simulink model "phase1_PRControl_CIM_Adapt"  (R2024a)
settings: Solver=VariableStepAuto  StartTime=0.0  StopTime=20  FixedStep=1e-6  MaxStep=1e-6  RelTol=1e-6
values from neighbouring files (symbols this model uses):
  alpha_adapt = 100    [phase1_PRControl_CIM_Adapt_init.m]
  Am0_can = sys0_ocf.A    [phase1_PRControl_CIM_Adapt_init.m]
  Bm1_can = sys1_ocf.B    [phase1_PRControl_CIM_Adapt_init.m]
  c_adapt = 0.1    [phase1_PRControl_CIM_Adapt_init.m]
  Cf = 22e-6    (= 2.2e-05)    [phase1_PRControl_CIM_Adapt_init.m]
  Cm0_can = sys0_ocf.C    [phase1_PRControl_CIM_Adapt_init.m]
  E = 1    [phase1_PRControl_CIM_Adapt_init.m]
  freq = 49.5    [phase1_PRControl_CIM_Adapt_init.m]
  L1 = 150e-6    (= 0.00015)    [phase1_PRControl_CIM_Adapt_init.m]
  L2g = L2+Lg    (= 0.00045)    [phase1_PRControl_CIM_Adapt_init.m]
  m_m1 = size(Bm1_can,2)    [phase1_PRControl_CIM_Adapt_init.m]
  n_m0 = size(Am0_can,1)    [phase1_PRControl_CIM_Adapt_init.m]
  p_e = size(E,1)    [phase1_PRControl_CIM_Adapt_init.m]
  PiInit = k0_adapt*eye(m_m1)    [phase1_PRControl_CIM_Adapt_init.m]
  Q_adapt = zeros(m_m1,1)    [phase1_PRControl_CIM_Adapt_init.m]
  R1 = 0.045    [phase1_PRControl_CIM_Adapt_init.m]
  R2g = R2+Rg    (= 0.135)    [phase1_PRControl_CIM_Adapt_init.m]
  Rd = 1    [phase1_PRControl_CIM_Adapt_init.m]
  Theta0 = w0^2    (= 98696.0440109)    [phase1_PRControl_CIM_Adapt_init.m]
  w = 2*pi*freq    (= 311.017672705)    [phase1_PRControl_CIM_Adapt_init.m]
undefined symbols (not defined in the file or in its folder): alfa, Am0, beta, Bm1, C_filter, Cm1, DiscIntNeverNeededParam, Dm1, Down, dt, n0, nu, Th_bar, Up
libraries: fl_lib x34, nesl_utility x23, ee_lib x9, spsSeriesRLCBranchLib x9, cstblocks x7, spsVoltageMeasurementLib x5, spsCurrentMeasurementLib x2, spsDCVoltageSourceLib x2, simulink x2, spsACVoltageSourceLib x1, spsControlledVoltageSourceLib x1, spsBreakerLib x1
(part 2 of 2)

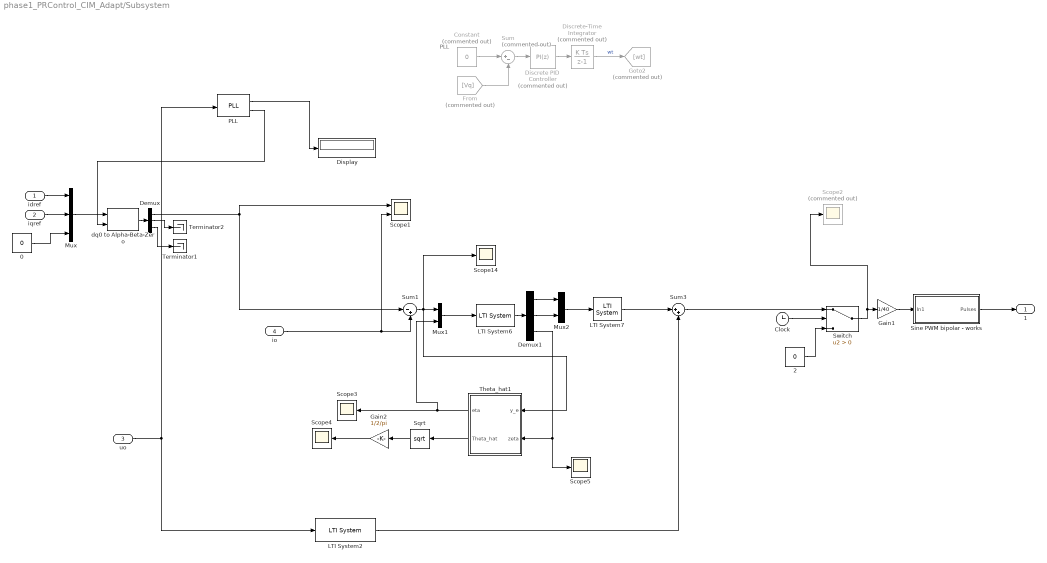
== system phase1_PRControl_CIM_Adapt/Subsystem ==
  note: PLL
  idref : Inport
  iqref : Inport  Port=2
  uo : Inport  Port=3
  io : Inport  Port=4
  0 : Constant  Value=0
  2 : Constant  Value=0
  Clock : Clock
  Constant : Constant  Commented=on  Value=0  SampleTime=10e-6
  Demux : Demux  Outputs=3
  Demux1 : Demux  Outputs=3
  Discrete PID Controller : slpidlib/PID Controller  Commented=on  Controller=PI  Form=Parallel  TimeDomain=Discrete-time  UseExternalTs=off  SampleTime=-1  IntegratorMethod=Forward Euler  FilterMethod=Forward Euler  ControllerParametersSource=internal  P=10  I=50000  UseKiTs=off  D=0  UseExternalDerivativeSource=off  N=100  UseFilter=on  TunerSelectOption=Transfer Function Based (PID Tuner App)  InitialConditionSource=internal  InitialConditionForIntegrator=0  InitialConditionForFilter=0  DifferentiatorICPrevScaledInput=0  ExternalReset=none  TrackingMode=off  Kt=1  LimitOutput=off  SatLimitsSource=internal  UpperSaturationLimit=inf  LowerSaturationLimit=-inf  LinearizeAsGain=off  AntiWindupMode=none  Kb=1  LimitIntegrator=off  UpperIntegratorSaturationLimit=inf  LowerIntegratorSaturationLimit=-inf  POutMin=[]  POutMax=[]  IOutMin=[]  IOutMax=[]  DOutMin=[]  DOutMax=[]  NOutMin=[]  NOutMax=[]  SumOutMin=[]  SumOutMax=[]  SaturationOutMin=[]  SaturationOutMax=[]  PParamMin=[]  PParamMax=[]  IParamMin=[]  IParamMax=[]  DParamMin=[]  DParamMax=[]  NParamMin=[]  NParamMax=[]  KbParamMin=[]  KbParamMax=[]  KtParamMin=[]  KtParamMax=[]  KbOutMin=[]  KbOutMax=[]  KtOutMin=[]  KtOutMax=[]  IntegratorOutMin=[]  IntegratorOutMax=[]  FilterOutMin=[]  FilterOutMax=[]  SumI1OutMin=[]  SumI1OutMax=[]  SumI2OutMin=[]  SumI2OutMax=[]  SumI3OutMin=[]  SumI3OutMax=[]  SumI4OutMin=[]  SumI4OutMax=[]  SumDOutMin=[]  SumDOutMax=[]  DifferentiatorOutMin=[]  DifferentiatorOutMax=[]  FilterDiffOutCoefMin=[]  FilterDiffOutCoefMax=[]  ReciprocalOutMin=[]  ReciprocalOutMax=[]  SumDenOutMin=[]  SumDenOutMax=[]  SumNumOutMin=[]  SumNumOutMax=[]  DivideOutMin=[]  DivideOutMax=[]  UdiffTsProdOutMin=[]  UdiffTsProdOutMax=[]  NTsProdOutMin=[]  NTsProdOutMax=[]  UintegralTsProdOutMin=[]  UintegralTsProdOutMax=[]  UngainTsProdOutMin=[]  UngainTsProdOutMax=[]  ClampingZeroOutDataTypeStr=Inherit: Inherit via back propagation  ClampingZeroOutMin=[]  ClampingZeroOutMax=[]  FilterDenConstantOutDataTypeStr=Inherit: Inherit via back propagation  FilterDenConstantOutMin=[]  FilterDenConstantOutMax=[]  PCopyOutDataTypeStr=Inherit: Inherit via back propagation  PCopyOutMin=[]  PCopyOutMax=[]  NCopyOutDataTypeStr=Inherit: Inherit via back propagation  NCopyOutMin=[]  NCopyOutMax=[]  IntegratorContinuousStateAttributes=''  IntegratorStateMustResolveToSignalObject=off  IntegratorRTWStateStorageClass=Auto  FilterContinuousStateAttributes=''  FilterStateMustResolveToSignalObject=off  FilterRTWStateStorageClass=Auto  ParallelPVariant=InternalParameters  IdealPVariant=Disabled  IVariant=InternalParameters  DVariant=Disabled  IntegratorVariant=Discrete  SatVariant=Disabled  AWVariant=Passthrough  PCopyVariant=Disabled  TRVariant=Disabled  FdbkBlocksVariant=Forward  IdealPFdbkVariant=Disabled  SatFdbkVariant=Disabled  DerivativeFilterVariant=Disabled  NVariant=Disabled  NCopyVariant=Disabled_SignalSpec  FilterICVariant=Disabled  IntegratorICVariant=InternalICs  ExternalResetVariant=Disabled  TRSumVariant=Passthrough  SumFdbkVariant=Disabled  SumVariant=Sum_PI  TsampFilterVariant=InternalTs  TsampNgainVariant=Passthrough  TsampIntegralVariant=Disabled_SignalSpec  ExternalSaturationOutDataTypeStr=Inherit: Same as second input  DerivativeSourceVariant=Disabled
      settings: LibrarySourceBlock=simulink/Discrete/Discrete PID Controller
  Discrete-Time Integrator : DiscreteIntegrator  Commented=on  SampleTime=-1  ICPrevOutput=DiscIntNeverNeededParam  ICPrevScaledInput=DiscIntNeverNeededParam
  Display : Display
  From : From  Commented=on  GotoTag=Vq
  Gain1 : Gain  Gain=1/40
  Gain2 : Gain  Gain=1/2/pi
  Goto2 : Goto  Commented=on  GotoTag=wt
  LTI System2 : cstblocks/LTI System  sys=Gfffilter  IC=[]  PadeOrder=0
  LTI System6 : cstblocks/LTI System  sys=Psi0dssss_min  IC=[]  PadeOrder=0
  LTI System7 : cstblocks/LTI System  sys=RI_tf  IC=[]  PadeOrder=0
  Mux : Mux  Inputs=3
  Mux1 : Mux  Inputs=2
  Mux2 : Mux  Inputs=2
  PLL : spsPLLLib/PLL  Fmin=49  Par_Init=[0, 50]  ParK=[180, 3200, 1]  TcD=1e-4  MaxRateChangeFreq=12  FilterCutOffFreq=25  Ts=0  AGC=on
      settings: LibrarySourceBlock=sps_lib/Control/PLL
  Scope1 : Scope  NumInputPorts=2
  Scope{3..5,14} (4 alike) : Scope
  Scope2 : Scope  Commented=on
  Sine PWM bipolar - works : Subsystem
  Sqrt : Sqrt
  Sum : Sum  Commented=on  Inputs=|+-
  Sum1 : Sum  Inputs=|-+
  Sum3 : Sum  Inputs=|++
  Switch : Switch  Criteria=u2 > Threshold  SaturateOnIntegerOverflow=off  InputSameDT=off
  Terminator1 : Terminator
  Terminator2 : Terminator
  Theta_hat1 : Subsystem
  dq0 to Alpha-Beta-Zero : spsdq0toAlphaBetaZeroLib/dq0 to Alpha-Beta-Zero  Alignment=90 degrees behind phase A axis
  1 : Outport
  wires:
  Constant/1 -> Sum/1
  From/1 -> Sum/2
  Sum/1 -> Discrete PID Controller/1
  Discrete PID Controller/1 -> Discrete-Time Integrator/1
  Discrete-Time Integrator/1 -> Goto2/1  "wt"
  Demux/1 -> Sum1/1, Scope1/1
  io/1 -> Scope1/2, Sum1/2
  Sine PWM bipolar - works/1(Pulses) -> 1/1
  Gain1/1 -> Sine PWM bipolar - works/1(In1)
  LTI System2/1 -> Sum3/2
  LTI System7/1 -> Sum3/1
  uo/1 -> LTI System2/1, PLL/1
  Mux/1 -> dq0 to Alpha-Beta-Zero/1
  0/1 -> Mux/3
  Demux/3 -> Terminator1/1
  Demux/2 -> Terminator2/1
  PLL/1 -> Display/1
  dq0 to Alpha-Beta-Zero/1 -> Demux/1
  PLL/2 -> dq0 to Alpha-Beta-Zero/2
  idref/1 -> Mux/1
  iqref/1 -> Mux/2
  2/1 -> Switch/3
  Clock/1 -> Switch/2
  Switch/1 -> Scope2/1, Gain1/1
  Sum3/1 -> Switch/1
  Mux1/1 -> LTI System6/1
  Demux1/1 -> Mux2/1
  LTI System6/1 -> Demux1/1
  Mux2/1 -> LTI System7/1
  Demux1/2 -> Mux2/2
  Theta_hat1/1(eta) -> Mux1/2, Scope3/1
  Theta_hat1/2(Theta_hat) -> Sqrt/1
  Sqrt/1 -> Gain2/1
  Sum1/1 -> Theta_hat1/1(y_e), Mux1/1, Scope14/1
  Demux1/3 -> Scope5/1, Theta_hat1/2(zeta)
  Gain2/1 -> Scope4/1

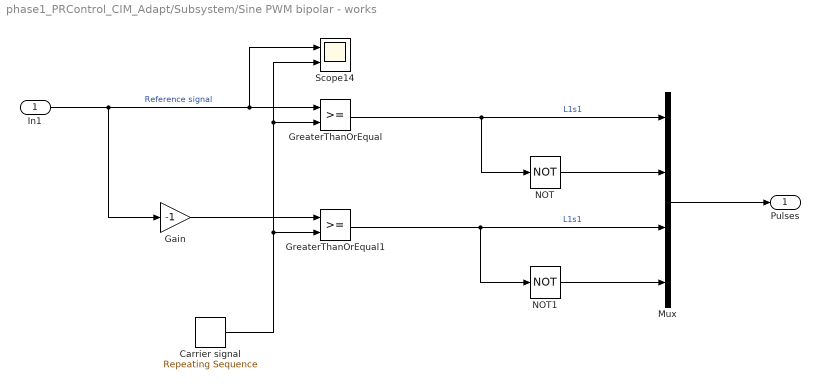
== system phase1_PRControl_CIM_Adapt/Subsystem/Sine PWM bipolar - works ==
  In1 : Inport
  Carrier signal : simulink/Sources/Repeating Sequence  rep_seq_t=[0 1/24000 1/12000]  rep_seq_y=[-1 1 -1]
  Gain : Gain  Gain=-1
  GreaterThanOrEqual : RelationalOperator  OutDataTypeStr=boolean  RndMeth=Simplest  InputSameDT=off
  GreaterThanOrEqual1 : RelationalOperator  OutDataTypeStr=boolean  RndMeth=Simplest  InputSameDT=off
  Mux : Mux
  NOT : Logic  Operator=NOT  IconShape=distinctive  AllPortsSameDT=off  OutDataTypeStr=boolean
  NOT1 : Logic  Operator=NOT  IconShape=distinctive  AllPortsSameDT=off  OutDataTypeStr=boolean
  Scope14 : Scope  NumInputPorts=2
  Pulses : Outport
  wires:
  Mux/1 -> Pulses/1
  In1/1 -> Scope14/1, GreaterThanOrEqual/1, Gain/1  "Reference signal"
  Carrier signal/1 -> Scope14/2, GreaterThanOrEqual/2, GreaterThanOrEqual1/2
  GreaterThanOrEqual/1 -> NOT/1, Mux/1  "L1s1"
  Gain/1 -> GreaterThanOrEqual1/1
  NOT/1 -> Mux/2
  GreaterThanOrEqual1/1 -> NOT1/1, Mux/3  "L1s1"
  NOT1/1 -> Mux/4

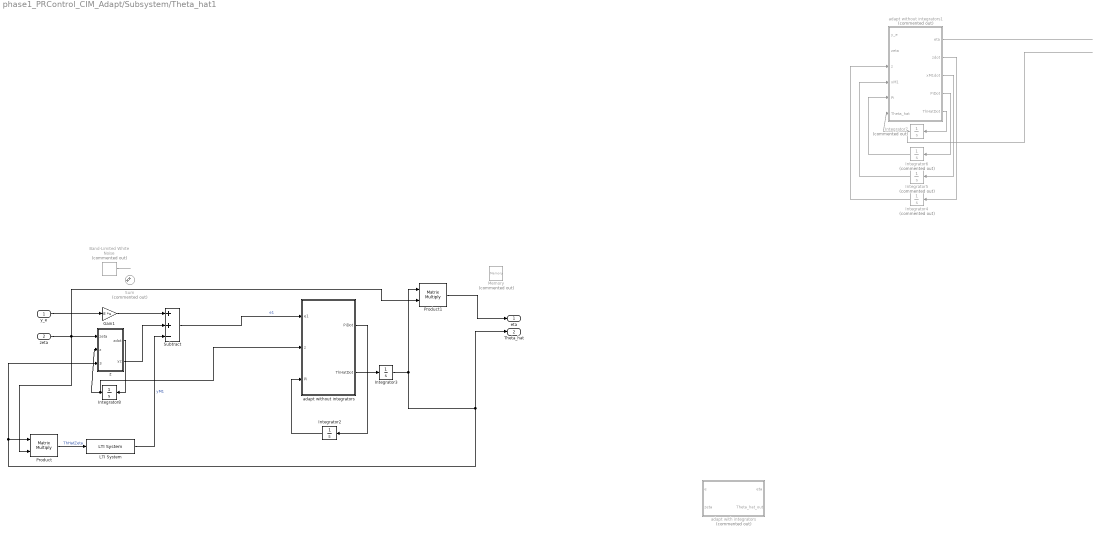
== system phase1_PRControl_CIM_Adapt/Subsystem/Theta_hat1 ==
  y_e : Inport
  zeta : Inport  Port=2
  Band-Limited White Noise : simulink/Sources/Band-Limited White Noise  Commented=on  Cov=[0.000001]  Ts=0.1  seed=[23341]
  Gain1 : Gain  Gain=E  Multiplication=Matrix(K*u)
  Integrator2 : Integrator  InitialCondition=PiInit
  Integrator3 : Integrator  InitialCondition=Theta0
  Integrator4 : Integrator  Commented=on  InitialCondition=ones(n_m0,m_m1)
  Integrator5 : Integrator  Commented=on  InitialCondition=zeros(n_m0,1)
  Integrator6 : Integrator  Commented=on  InitialCondition=PiInit
  Integrator7 : Integrator  Commented=on  InitialCondition=Th_bar
  Integrator8 : Integrator  InitialCondition=zeros(n_m0,m_m1)
  LTI System : cstblocks/LTI System  sys=ss(Am0_can,Bm1_can,Cm0_can, zeros(p_e,m_m1))  IC=zeros(n_m0,1)  PadeOrder=0
  Memory : Memory  Commented=on
  Product : Product  Multiplication=Matrix(*)
  Product1 : Product  Multiplication=Matrix(*)
  Subtract : Sum  Inputs=++-
  Sum : Sum  Commented=on  Inputs=++|
  adapt with integrators : MATLAB Function  Commented=on  TreatAsAtomicUnit=on
  adapt without integrators : MATLAB Function
  adapt without integrators1 : MATLAB Function  Commented=on
  z : MATLAB Function
  eta : Outport
  Theta_hat : Outport  Port=2
  wires:
  zeta/1 -> Product1/2, Product/2, z/1(zeta)
  adapt without integrators/1(PiDot) -> Integrator2/1
  Integrator2/1 -> adapt without integrators/3(Pi)
  adapt without integrators/2(ThHatDot) -> Integrator3/1
  Integrator3/1 -> Product1/1, Theta_hat/1, z/3(Theta_hat), Product/1
  adapt without integrators1/3(xM1dot) -> Integrator5/1
  Integrator5/1 -> adapt without integrators1/4(xM1)
  Integrator7/1 -> adapt without integrators1/6(Theta_hat)
  adapt without integrators1/1(eta) -> ?
  adapt without integrators1/5(ThHatDot) -> Integrator7/1
  ? -> adapt without integrators1/1(y_e)
  ? -> adapt without integrators1/2(zeta)
  adapt without integrators1/2(zdot) -> Integrator4/1
  Integrator4/1 -> adapt without integrators1/3(z)
  adapt without integrators1/4(PiDot) -> Integrator6/1
  Integrator6/1 -> adapt without integrators1/5(Pi)
  z/1(zdot) -> Integrator8/1
  Integrator8/1 -> adapt without integrators/2(z), z/2(z)
  Product/1 -> LTI System/1  "ThHatZeta"
  LTI System/1 -> Subtract/3  "yM1"
  y_e/1 -> Gain1/1
  z/2(yz) -> Subtract/2
  Subtract/1 -> adapt without integrators/1(e1)  "e1"
  Product1/1 -> eta/1
  Gain1/1 -> Subtract/1
  Band-Limited White Noise/1 -> ?

== matlab function phase1_PRControl_CIM_Adapt/Subsystem/Theta_hat1/adapt with integrators ==
  settings: updateMethod=DISCRETE  sampleTime=dt
  data: e input; eta output; zeta input; Theta_hat_out output; Am0 parameter; Bm1 parameter; Cm1 parameter; Dm1 parameter; dt parameter; n0 parameter; nu parameter; c_adapt parameter; alpha_adapt parameter; PiInit parameter; Q_adapt parameter
function [eta,Theta_hat_out] = fcn(e,zeta,Am0,Bm1, Cm1, Dm1,dt, n0, nu,c_adapt, alpha_adapt,PiInit,Q_adapt)
%#codegen

persistent Theta_hat z xM1 Pi

nu = 2;     % <- FIXED here for this model
n0 = 5;     % <- order of Am0

if isempty(Theta_hat)

    Pi=PiInit;
    Theta_hat = [100;100];
    z = zeros(n0,nu);
    xM1 = zeros(n0,1);
end

% --- 1) z-filter:  ż = A0 z + B1 ζ ---
zdot = Am0*z + Bm1*zeta;
z    = z + dt*zdot;

% --- 2) M1(Θ̂) ζ realization ---
xM1dot = Am0*xM1 + Bm1*(Theta_hat*zeta);   % 5×1 + 5×2*(2×1)
xM1    = xM1 + dt*xM1dot;
yM1    = Cm1*xM1 + Dm1*(Theta_hat*zeta);   % scalar

% --- 3) e1 = e + C0 z Θ̂ − M1 Θ̂ ζ ---
c0z = Cm1*z;                     % 1×5 * 5×2 = 1×2
e1  = [1 0]*e + c0z*Theta_hat - yM1;  % scalar

% --- 4) NLS adaptation Θ̂̇, Π̇ ---
N = c_adapt + c0z*c0z' + c0z*Pi*c0z';
if N < 1e-6
    N = 1e-6;
end

PiDot = -Pi*(c0z')*c0z*Pi/N + 2*alpha_adapt*Pi/N;
Pi    = Pi + dt*PiDot;
Pi    = 0.5*(Pi + Pi.');        % keep symmetric

ThetaDot  = Pi*(c0z')*e1/N + Q_adapt;
Theta_hat = Theta_hat + dt*ThetaDot;

% --- 5) output η = Θ̂ ζ ---
eta = Theta_hat*zeta;
Theta_hat_out = Theta_hat;

== matlab function phase1_PRControl_CIM_Adapt/Subsystem/Theta_hat1/adapt without integrators ==
  settings: updateMethod=CONTINUOUS  sampleTime=dt
  data: Cm0_can parameter; c_adapt parameter; alpha_adapt parameter; Q_adapt parameter; e1 input; z input; Pi input; PiDot output; ThHatDot output
function [PiDot,ThHatDot] = fcn(Cm0_can,c_adapt, alpha_adapt,Q_adapt,e1, z, Pi)


% N = c_adapt + Cm1z*Cm1z' + Cm1z*Pi*Cm1z';
N_adapt = c_adapt + (Cm0_can*z)*(Cm0_can*z)' + (Cm0_can*z)*Pi*(Cm0_can*z)';
% PiDot = -Pi*(Cm1z')*Cm1z*Pi/N + 2*alpha_adapt*Pi/N;
PiDot=-Pi*(Cm0_can*z)'*(Cm0_can*z)*Pi/N_adapt+2*alpha_adapt*Pi/N_adapt;

% ThetaDot = -Pi*(Cm1z')*e1/N + Q_adapt;
ThHatDot = -Pi*(Cm0_can*z)'*e1/N_adapt+Q_adapt;

== matlab function phase1_PRControl_CIM_Adapt/Subsystem/Theta_hat1/adapt without integrators1 ==
  settings: updateMethod=CONTINUOUS  sampleTime=dt
  data: y_e input; eta output; zeta input; Am0_can parameter; Bm1_can parameter; Cm0_can parameter; c_adapt parameter; alpha_adapt parameter; Q_adapt parameter; z input; xM1 input; Pi input; Theta_hat input; zdot output; xM1dot output; PiDot output; ThHatDot output; E parameter
function [eta,zdot,xM1dot,PiDot,ThHatDot] = fcn(y_e,zeta,Am0_can,Bm1_can, Cm0_can,c_adapt, alpha_adapt,Q_adapt, z, xM1, Pi, Theta_hat, E)

zdot = Am0_can*z + Bm1_can*zeta;
yz=Cm0_can*z*Theta_hat;
xM1dot = Am0_can*xM1 + Bm1_can*(Theta_hat*zeta);   
yM1    = Cm0_can*xM1;   

% Cm1z = Cm0_can*z;                    
e   = E*y_e;
e1  = e + yz - yM1; 

% N = c_adapt + Cm1z*Cm1z' + Cm1z*Pi*Cm1z';
N_adapt = c_adapt + (Cm0_can*z)*(Cm0_can*z)' + (Cm0_can*z)*Pi*(Cm0_can*z)';
% PiDot = -Pi*(Cm1z')*Cm1z*Pi/N + 2*alpha_adapt*Pi/N;
PiDot=-Pi*(Cm0_can*z)'*(Cm0_can*z)*Pi/N_adapt+2*alpha_adapt*Pi/N_adapt;

% ThetaDot = -Pi*(Cm1z')*e1/N + Q_adapt;
ThHatDot = -Pi*(Cm0_can*z)'*e1/N_adapt+Q_adapt;
eta = Theta_hat*zeta;

== matlab function phase1_PRControl_CIM_Adapt/Subsystem/Theta_hat1/z ==
  settings: updateMethod=CONTINUOUS  sampleTime=dt
  data: zdot output; yz output; zeta input; Am0_can parameter; Bm1_can parameter; Cm0_can parameter; z input; Theta_hat input
function [zdot,yz] = fcn(zeta,Am0_can,Bm1_can, Cm0_can, z, Theta_hat)

zdot = Am0_can*z + Bm1_can*zeta;
yz=Cm0_can*z*Theta_hat;
